simulink model "sl_quadrotor_orgional"  (Simulink 7.8)
settings: Solver=ode45  StartTime=0.0  StopTime=20  MaxStep=0.1  RelTol=1e-3
InitFcn:
  | % load parameters of the default quadrotor
  | disp('Quadrotor parameters loaded by InitFcn')
  | mdl_quadcopter
undefined symbols (not defined in the file or in its folder): quad
libraries: roblocks x3, simulink x1
settings Model: Creator=corkep  LastModifiedBy=deep
settings DebuggingCC: StrictBusMsg=Warning

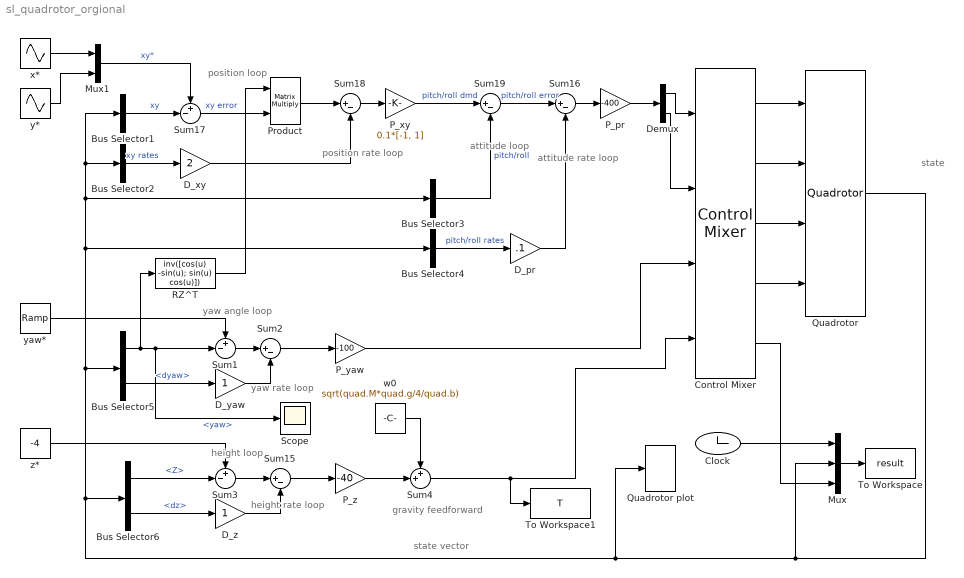
== system sl_quadrotor_orgional ==
  note: state vector
  note: gravity feedforward
  note: attitude rate
      | loop
  note: attitude
      | loop
  note: position rate
      | loop
  note: position
      | loop
  note: yaw rate
      | loop
  note: yaw angle
      | loop
  note: height rate
      | loop
  note: height
      | loop
  note: state
  Bus Selector1 : BusSelector  OutputSignals=X,Y  OutputAsBus=on
  Bus Selector2 : BusSelector  OutputSignals=dx,dy  OutputAsBus=on
  Bus Selector3 : BusSelector  OutputSignals=pitch,roll  OutputAsBus=on
  Bus Selector4 : BusSelector  OutputSignals=dpitch,droll  OutputAsBus=on
  Bus Selector5 : BusSelector  OutputSignals=yaw,dyaw
  Bus Selector6 : BusSelector  OutputSignals=Z,dz
  Clock : Clock
  Control Mixer : roblocks/Dynamics/Control Mixer
  D_pr : Gain  Gain=.1
  D_xy : Gain  Gain=2
  D_yaw : Gain
  D_z : Gain
  Demux : Demux  Outputs=2
  Mux : Mux  Inputs=3
  Mux1 : Mux  Inputs=2
  P_pr : Gain  Gain=-400
  P_xy : Gain  Gain=0.1*[-1, 1]
  P_yaw : Gain  Gain=-100
  P_z : Gain  Gain=-40
  Product : Product  Multiplication=Matrix(*)  RndMeth=Zero
  Quadrotor : roblocks/Dynamics/Quadrotor
  Quadrotor plot : roblocks/Robot Graphics/Quadrotor plot
  RZ^T : MATLABFcn  MATLABFcn=inv([cos(u) -sin(u); sin(u) cos(u)])  OutputDimensions=[2 2]  Output1D=off
  Scope : Scope
      settings: TimeRange=20  YMin=-0.0015  YMax=0.003000000000000001
  Sum1 : Sum  Inputs=+-|
  Sum{2,15..16,18..19} (5 alike) : Sum  Inputs=|+-
  Sum17 : Sum  Inputs=+-|
  Sum3 : Sum  Inputs=+-|
  Sum4 : Sum  Inputs=++|
  To Workspace : ToWorkspace  VariableName=result  SampleTime=-1  SaveFormat=Array
  To Workspace1 : ToWorkspace  VariableName=T  SampleTime=-1  SaveFormat=Array
  w0 : Constant  Value=sqrt(quad.M*quad.g/4/quad.b)  SampleTime=0
  x* : Sin  Frequency=2*pi*.125  Phase=-pi/2  SampleTime=0
  y* : Sin  Frequency=2*pi*.125  SampleTime=0
  yaw* : simulink/Sources/Ramp  slope=0.2  start=2  X0=0
  z* : Constant  Value=-4  SampleTime=0
  wires:
  Control Mixer/1 -> Quadrotor/1
  Control Mixer/4 -> Quadrotor/4
  w0/1 -> Sum4/1
  Sum15/1 -> P_z/1
  P_z/1 -> Sum4/2
  Quadrotor/1 -> Bus Selector6/1, Bus Selector4/1, Bus Selector3/1, Bus Selector1/1, Bus Selector2/1, Bus Selector5/1, Quadrotor plot/1, Mux/2
  x*/1 -> Mux1/1
  y*/1 -> Mux1/2
  Bus Selector1/1 -> Sum17/2  "xy"
  Mux1/1 -> Sum17/1  "xy*"
  Bus Selector2/1 -> D_xy/1  "xy rates"
  D_xy/1 -> Sum18/2
  P_xy/1 -> Sum19/1  "pitch/roll dmd"
  Bus Selector3/1 -> Sum19/2  "pitch/roll"
  Bus Selector4/1 -> D_pr/1  "pitch/roll rates"
  Sum19/1 -> Sum16/1  "pitch/roll error"
  Sum16/1 -> P_pr/1
  P_pr/1 -> Demux/1
  P_yaw/1 -> Control Mixer/3
  Bus Selector5/1 -> RZ^T/1, Sum1/2, Scope/1  "<yaw>"
  Sum2/1 -> P_yaw/1
  Bus Selector6/1 -> Sum3/2  "<Z>"
  z*/1 -> Sum3/1
  Bus Selector5/2 -> D_yaw/1  "<dyaw>"
  Sum3/1 -> Sum15/1
  Bus Selector6/2 -> D_z/1  "<dz>"
  D_z/1 -> Sum15/2
  D_pr/1 -> Sum16/2
  Demux/2 -> Control Mixer/2
  D_yaw/1 -> Sum2/2
  Sum4/1 -> To Workspace1/1, Control Mixer/4
  Sum1/1 -> Sum2/1
  Mux/1 -> To Workspace/1
  Clock/1 -> Mux/1
  Control Mixer/5 -> Mux/3
  Sum18/1 -> P_xy/1
  yaw*/1 -> Sum1/1
  Product/1 -> Sum18/1
  Sum17/1 -> Product/2  "xy error"
  RZ^T/1 -> Product/1
  Demux/1 -> Control Mixer/1
  Control Mixer/3 -> Quadrotor/3
  Control Mixer/2 -> Quadrotor/2
